simulink model "Modelo_motor_blockset"  (R2023b)
settings: Solver=VariableStepAuto  StartTime=0.0  StopTime=4  RelTol=1e-3
libraries: spsAsynchronousMachineSIUnitsLib x5, simulink x5, spsThreePhaseVIMeasurementLib x5, spsPWMGenerator2LevelLib x4, spsUniversalBridgeLib x4, spsDCVoltageSourceLib x3, spsControlledVoltageSourceLib x1, spsGroundLib x1, spsSVPWMGenerator2LevelLib x1, spsThreePhaseProgrammableVoltageSourceLib x1, sps_lib x1
settings Model: Creator=Jorge  LastModifiedBy=Jorge

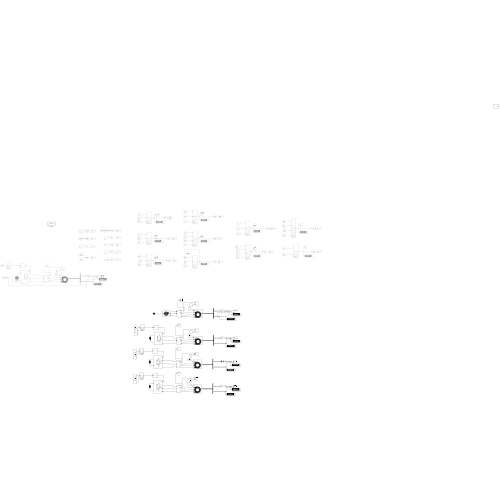
[thumbnail: Simulink's stored preview of the top-level diagram]
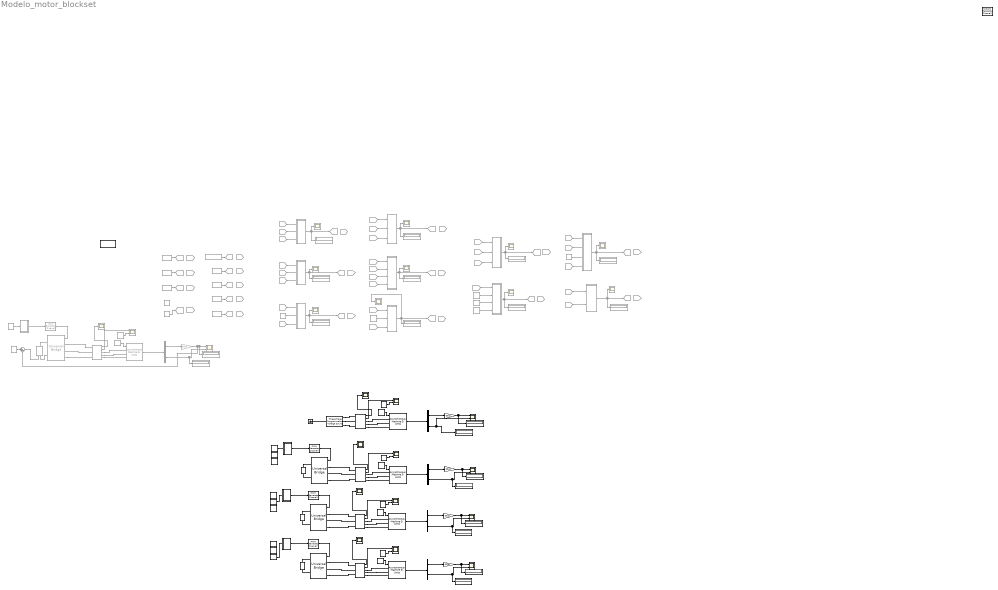
== system Modelo_motor_blockset ==
  120 : Constant  Commented=on  Value=120
  Asynchronous Machine SI Units : spsAsynchronousMachineSIUnitsLib/Asynchronous Machine SI Units  RotorType=Squirrel-cage  PresetModel=No  MechanicalLoad=Torque Tm  ShowDetailedParameters=on  ReferenceFrame=Rotor  Units=SI  MeasurementBus=off  NominalParameters=[950 220 60]  VoltageRatio=1  Stator=[0.2 3/(2*pi*60)]  Rotor=[1.3 2/(2*pi*60)]  Cage1=[0.4155 0.002066]  Cage2=[0.4168 0.0003495]  Lm=28/(2*pi*60)  Mechanical=[0.1 0.0 4]  PolePairs=2  InitialConditions=[1 0 0 0 0 0 120 -120]  SimulateSaturation=off  Saturation=[14.03593122, 27.81365428, 53.79336849, 72.68890987, 97.98006896, 148.6815601, 215.7428561, 302.9841135, 428.7778367 ; 230, 322, 414, 460, 506, 552, 598, 644, 690]  LoadFlowParameters=1492000  TsPowergui=0  TsBlock=-1  IterativeModel=Trapezoidal non iterative  IterativeDiscreteModel=Trapezoidal non iterative  Pmec=866
  Asynchronous Machine SI Units1 : spsAsynchronousMachineSIUnitsLib/Asynchronous Machine SI Units  RotorType=Squirrel-cage  PresetModel=No  MechanicalLoad=Torque Tm  ShowDetailedParameters=on  ReferenceFrame=Rotor  Units=SI  MeasurementBus=off  NominalParameters=[907 220/sqrt(3) 60]  VoltageRatio=1  Stator=[0.2 3/(2*pi*60)]  Rotor=[1.3 2/(2*pi*60)]  Cage1=[0.4155 0.002066]  Cage2=[0.4168 0.0003495]  Lm=28/(2*pi*60)  Mechanical=[0.1 0.0 4]  PolePairs=2  InitialConditions=[1 0 0 0 0 0 -120 120]  SimulateSaturation=off  Saturation=[14.03593122, 27.81365428, 53.79336849, 72.68890987, 97.98006896, 148.6815601, 215.7428561, 302.9841135, 428.7778367 ; 230, 322, 414, 460, 506, 552, 598, 644, 690]  LoadFlowParameters=1492000  TsPowergui=0  TsBlock=-1  IterativeModel=Trapezoidal non iterative  IterativeDiscreteModel=Trapezoidal non iterative  Pmec=866
  Asynchronous Machine SI Units2 : spsAsynchronousMachineSIUnitsLib/Asynchronous Machine SI Units  Commented=on  RotorType=Squirrel-cage  PresetModel=No  MechanicalLoad=Torque Tm  ShowDetailedParameters=on  ReferenceFrame=Rotor  Units=SI  MeasurementBus=off  NominalParameters=[907 220/sqrt(3) 60]  VoltageRatio=1  Stator=[0.2 3/(2*pi*60)]  Rotor=[1.3 2/(2*pi*60)]  Cage1=[0.4155 0.002066]  Cage2=[0.4168 0.0003495]  Lm=28/(2*pi*60)  Mechanical=[0.1 0.0 4]  PolePairs=2  InitialConditions=[1 0 0 0 0 0 -120 120]  SimulateSaturation=off  Saturation=[14.03593122, 27.81365428, 53.79336849, 72.68890987, 97.98006896, 148.6815601, 215.7428561, 302.9841135, 428.7778367 ; 230, 322, 414, 460, 506, 552, 598, 644, 690]  LoadFlowParameters=1492000  TsPowergui=0  TsBlock=-1  IterativeModel=Trapezoidal non iterative  IterativeDiscreteModel=Trapezoidal non iterative  Pmec=866
  Asynchronous Machine SI Units3 : spsAsynchronousMachineSIUnitsLib/Asynchronous Machine SI Units  RotorType=Squirrel-cage  PresetModel=No  MechanicalLoad=Torque Tm  ShowDetailedParameters=on  ReferenceFrame=Rotor  Units=SI  MeasurementBus=off  NominalParameters=[907 220/sqrt(3) 60]  VoltageRatio=1  Stator=[0.2 3/(2*pi*60)]  Rotor=[1.3 2/(2*pi*60)]  Cage1=[0.4155 0.002066]  Cage2=[0.4168 0.0003495]  Lm=28/(2*pi*60)  Mechanical=[0.1 0.0 4]  PolePairs=2  InitialConditions=[1 0 0 0 0 0 -120 120]  SimulateSaturation=off  Saturation=[14.03593122, 27.81365428, 53.79336849, 72.68890987, 97.98006896, 148.6815601, 215.7428561, 302.9841135, 428.7778367 ; 230, 322, 414, 460, 506, 552, 598, 644, 690]  LoadFlowParameters=1492000  TsPowergui=0  TsBlock=-1  IterativeModel=Trapezoidal non iterative  IterativeDiscreteModel=Trapezoidal non iterative  Pmec=866
  Asynchronous Machine SI Units4 : spsAsynchronousMachineSIUnitsLib/Asynchronous Machine SI Units  RotorType=Squirrel-cage  PresetModel=No  MechanicalLoad=Torque Tm  ShowDetailedParameters=on  ReferenceFrame=Rotor  Units=SI  MeasurementBus=off  NominalParameters=[907 220/sqrt(3) 60]  VoltageRatio=1  Stator=[0.2 3/(2*pi*60)]  Rotor=[1.3 2/(2*pi*60)]  Cage1=[0.4155 0.002066]  Cage2=[0.4168 0.0003495]  Lm=28/(2*pi*60)  Mechanical=[0.1 0.0 4]  PolePairs=2  InitialConditions=[1 0 0 0 0 0 -120 120]  SimulateSaturation=off  Saturation=[14.03593122, 27.81365428, 53.79336849, 72.68890987, 97.98006896, 148.6815601, 215.7428561, 302.9841135, 428.7778367 ; 230, 322, 414, 460, 506, 552, 598, 644, 690]  LoadFlowParameters=1492000  TsPowergui=0  TsBlock=-1  IterativeModel=Trapezoidal non iterative  IterativeDiscreteModel=Trapezoidal non iterative  Pmec=866
  Bus Selector{,1,3..4} (4 alike) : BusSelector  OutputSignals=Mechanical.Rotor speed (wm),Mechanical.Electromagnetic torque Te (N*m)
  Bus Selector2 : BusSelector  Commented=on  OutputSignals=Mechanical.Rotor speed (wm),Mechanical.Electromagnetic torque Te (N*m)
  Constant : Constant  Commented=on
  Constant1 : Constant  Commented=on
  Constant{6,10,16,21} (4 alike) : Constant  Value=4.94
  Constant11 : Constant  Commented=on  Value=60
  Constant12 : Constant  Commented=on  Value=4.74
  Constant13 : Constant  Commented=on  Value=1746
  Constant14 : Constant  Value=40
  Constant15 : Constant  Value=20
  Constant17 : Constant  Value=40
  Constant18 : Constant  Value=20
  Constant19 : Constant  Value=60
  Constant2 : Constant  Commented=on  Value=2
  Constant{5,9,20,25} (4 alike) : Constant  Value=4.74
  Constant22 : Constant  Value=40
  Constant23 : Constant  Value=20
  Constant24 : Constant  Value=60
  Constant3 : Constant  Commented=on  Value=0.03
  Constant4 : Constant  Commented=on  Value=60
  Constant7 : Constant  Value=60
  Constant8 : Constant  Commented=on  Value=4.94
  Controlled Voltage Source1 : spsControlledVoltageSourceLib/Controlled Voltage Source  Commented=on  Initialize=on  Source_Type=DC  Amplitude=220  Phase=0  Frequency=0  Measurements=None
  DC Voltage Source : spsDCVoltageSourceLib/DC Voltage Source  Amplitude=220*(sqrt(3)/sqrt(2))*0.945  Measurements=Voltage
  DC Voltage Source1 : spsDCVoltageSourceLib/DC Voltage Source  Amplitude=220*(sqrt(3)/sqrt(2))*0.945  Measurements=Voltage
  DC Voltage Source2 : spsDCVoltageSourceLib/DC Voltage Source  Amplitude=220*(sqrt(3)/sqrt(2))*0.945  Measurements=Voltage
  Display{,1..9,14..15} (12 alike) : Display  Commented=on
  Display{10..13,16..19} (8 alike) : Display
  From{,3,12,34} (4 alike) : From  Commented=on  GotoTag=V1
  From1 : From  Commented=on  GotoTag=R1
  From10 : From  Commented=on  GotoTag=I2
  From11 : From  Commented=on  GotoTag=I1
  From13 : From  Commented=on  GotoTag=R1
  From{2,14,33,37} (4 alike) : From  Commented=on  GotoTag=X1
  From{6,15,25,29} (4 alike) : From  Commented=on  GotoTag=R2
  From16 : From  Commented=on  GotoTag=X2
  From{5,17,21,26,30} (5 alike) : From  Commented=on  GotoTag=S
  From18 : From  Commented=on  GotoTag=f
  From19 : From  Commented=on  GotoTag=p
  From20 : From  Commented=on  GotoTag=Ns
  From22 : From  Commented=on  GotoTag=N
  From23 : From  Commented=on  GotoTag=Ns
  From24 : From  Commented=on  GotoTag=I2
  From27 : From  Commented=on  GotoTag=Pag
  From28 : From  Commented=on  GotoTag=I2
  From31 : From  Commented=on  GotoTag=Pmec
  From32 : From  Commented=on  GotoTag=Xm
  From35 : From  Commented=on  GotoTag=Vth
  From36 : From  Commented=on  GotoTag=Xm
  From38 : From  Commented=on  GotoTag=R1
  From39 : From  Commented=on  GotoTag=Rth
  From4 : From  Commented=on  GotoTag=X2
  From40 : From  Commented=on  GotoTag=Ns
  From41 : From  Commented=on  GotoTag=ws
  From42 : From  Commented=on  GotoTag=Pag
  From43 : From  Commented=on  GotoTag=ws
  From44 : From  Commented=on  GotoTag=T
  From7 : From  Commented=on  GotoTag=f
  From8 : From  Commented=on  GotoTag=p
  From9 : From  Commented=on  GotoTag=Xm
  Gain{,2..4} (4 alike) : Gain  Gain=60/pi
  Gain1 : Gain  Commented=on  Gain=60/pi
  Goto : Goto  Commented=on  GotoTag=V1
  Goto1 : Goto  Commented=on  GotoTag=f
  Goto10 : Goto  Commented=on  GotoTag=I1
  Goto11 : Goto  Commented=on  GotoTag=Ns
  Goto12 : Goto  Commented=on  GotoTag=N
  Goto13 : Goto  Commented=on  GotoTag=Pag
  Goto14 : Goto  Commented=on  GotoTag=Pmec
  Goto15 : Goto  Commented=on  GotoTag=Vth
  Goto16 : Goto  Commented=on  GotoTag=Rth
  Goto17 : Goto  Commented=on  GotoTag=ws
  Goto18 : Goto  Commented=on  GotoTag=T
  Goto2 : Goto  Commented=on  GotoTag=p
  Goto3 : Goto  Commented=on  GotoTag=R1
  Goto4 : Goto  Commented=on  GotoTag=X1
  Goto5 : Goto  Commented=on  GotoTag=R2
  Goto6 : Goto  Commented=on  GotoTag=X2
  Goto7 : Goto  Commented=on  GotoTag=Xm
  Goto8 : Goto  Commented=on  GotoTag=S
  Goto9 : Goto  Commented=on  GotoTag=I2
  Ground : spsGroundLib/Ground  LConnTagsString=a
  PWM Generator (2-Level) : spsPWMGenerator2LevelLib/PWM Generator (2-Level)  ModulatorType=Three-phase bridge (6 pulses)  ModulatorMode=Unsynchronized  Fc=60*39  Pc=0  nF=27  MinMax="[ -1  1 ]"  SamplingTechnique=Natural  ModulatingSignals=off  m=0.8  Freq=60  Phase=0  Ts=0  ShowCarrierOutport=off
  PWM Generator (2-Level)1 : spsPWMGenerator2LevelLib/PWM Generator (2-Level)  Commented=on  ModulatorType=Three-phase bridge (6 pulses)  ModulatorMode=Unsynchronized  Fc=60*39  Pc=0  nF=27  MinMax="[ -1  1 ]"  SamplingTechnique=Natural  ModulatingSignals=off  m=0.8  Freq=60  Phase=0  Ts=0  ShowCarrierOutport=off
  PWM Generator (2-Level)2 : spsPWMGenerator2LevelLib/PWM Generator (2-Level)  ModulatorType=Three-phase bridge (6 pulses)  ModulatorMode=Unsynchronized  Fc=60*39  Pc=0  nF=27  MinMax="[ -1  1 ]"  SamplingTechnique=Natural  ModulatingSignals=off  m=0.8  Freq=60  Phase=0  Ts=0  ShowCarrierOutport=off
  PWM Generator (2-Level)3 : spsPWMGenerator2LevelLib/PWM Generator (2-Level)  ModulatorType=Three-phase bridge (6 pulses)  ModulatorMode=Unsynchronized  Fc=60*39  Pc=0  nF=27  MinMax="[ -1  1 ]"  SamplingTechnique=Natural  ModulatingSignals=off  m=0.8  Freq=60  Phase=0  Ts=0  ShowCarrierOutport=off
  Pi : Constant  Commented=on  Value=pi  OutDataTypeStr=Inherit: Inherit via back propagation
  R1 : Constant  Commented=on  Value=0.2
  R2 : Constant  Commented=on  Value=1.3
  SVPWM Generator (2-Level) : spsSVPWMGenerator2LevelLib/SVPWM Generator (2-Level)  InputType=Internally generated  SwitchingPattern=Pattern #1  Fc=2000  ParUref=[1 0 60]  Ts=0
  Scope{,1..9,17} (11 alike) : Scope  Commented=on
  Scope{10..11,13,15,19,21..22,24} (8 alike) : Scope  NumInputPorts=2
  Scope{12,14,20,23} (4 alike) : Scope
  Scope16 : Scope  Commented=on  NumInputPorts=2
  Scope18 : Scope  Commented=on  NumInputPorts=2
  Sinal : Subsystem
  Sinal1 : Subsystem  Commented=on
  Sinal2 : Subsystem
  Sinal3 : Subsystem
  Subsystem : Subsystem  Commented=on
  Subsystem1 : Subsystem  Commented=on
  Subsystem2 : Subsystem  Commented=on
  Subsystem3 : Subsystem  Commented=on
  Subsystem4 : Subsystem  Commented=on
  Subsystem5 : Subsystem  Commented=on
  Subsystem6 : Subsystem  Commented=on
  Subsystem7 : Subsystem  Commented=on
  Subsystem8 : Subsystem  Commented=on
  Subsystem9 : Subsystem  Commented=on
  Sum : Sum  Commented=on  Inputs=|+-
  Three-Phase Programmable Voltage Source : spsThreePhaseProgrammableVoltageSourceLib/Three-Phase Programmable Voltage Source  PositiveSequence=[220/sqrt(2) 0 60]  VariationEntity=None  VariationType=Table of time-amplitude pairs  VariationTypeAlt=Step  VariationStep=0.5  VariationRate=10  VariationMagnitude=0.3  VariationFrequency=2  VariationTiming=[1 2]  VariationPhaseA=off  Amplitudes=[1 0.8 1.2 1.0]  TimeValues=[0 0.1 0.15 0.2]  HarmonicGeneration=off  HarmonicA=[3 0.2 -25 0]  HarmonicB=[2 0.15 35 2]  Timing="[0.05  3]"  BusType=swing  Pref=0  Qref=0  Qmin=-inf  Qmax=inf
  Three-Phase V-I Measurement{,1,3..4} (4 alike) : spsThreePhaseVIMeasurementLib/Three-Phase V-I Measurement  VoltageMeasurement=phase-to-phase  SetLabelV=off  LabelV=Vabc  Vpu=off  VpuLL=off  CurrentMeasurement=yes  SetLabelI=off  LabelI=Iabc  Ipu=off  Pbase=100e6  Vbase=500e3  OutputType=Complex  PhasorSimulation=off  PSBequivalent=0
  Three-Phase V-I Measurement2 : spsThreePhaseVIMeasurementLib/Three-Phase V-I Measurement  Commented=on  VoltageMeasurement=phase-to-phase  SetLabelV=off  LabelV=Vabc  Vpu=off  VpuLL=off  CurrentMeasurement=yes  SetLabelI=off  LabelI=Iabc  Ipu=off  Pbase=100e6  Vbase=500e3  OutputType=Complex  PhasorSimulation=off  PSBequivalent=0
  Universal Bridge : spsUniversalBridgeLib/Universal Bridge  Arms=3  SnubberResistance=1e5  SnubberCapacitance=inf  Device=IGBT / Diodes  Ron=1e-3  Lon=0  ForwardVoltages="[  0  0  ]"  ForwardVoltage=0  GTOparameters=[ 10e-6 , 20e-6 ]  IGBTparameters=[ 1e-6 , 2e-6 ]  Measurements=None  Measurements_2=None  converterType=Rectifier
  Universal Bridge1 : spsUniversalBridgeLib/Universal Bridge  Commented=on  Arms=3  SnubberResistance=1e5  SnubberCapacitance=inf  Device=IGBT / Diodes  Ron=1e-3  Lon=0  ForwardVoltages="[  0  0  ]"  ForwardVoltage=0  GTOparameters=[ 10e-6 , 20e-6 ]  IGBTparameters=[ 1e-6 , 2e-6 ]  Measurements=None  Measurements_2=None  converterType=Rectifier
  Universal Bridge2 : spsUniversalBridgeLib/Universal Bridge  Arms=3  SnubberResistance=1e5  SnubberCapacitance=inf  Device=IGBT / Diodes  Ron=1e-3  Lon=0  ForwardVoltages="[  0  0  ]"  ForwardVoltage=0  GTOparameters=[ 10e-6 , 20e-6 ]  IGBTparameters=[ 1e-6 , 2e-6 ]  Measurements=None  Measurements_2=None  converterType=Rectifier
  Universal Bridge3 : spsUniversalBridgeLib/Universal Bridge  Arms=3  SnubberResistance=1e5  SnubberCapacitance=inf  Device=IGBT / Diodes  Ron=1e-3  Lon=0  ForwardVoltages="[  0  0  ]"  ForwardVoltage=0  GTOparameters=[ 10e-6 , 20e-6 ]  IGBTparameters=[ 1e-6 , 2e-6 ]  Measurements=None  Measurements_2=None  converterType=Rectifier
  V1 : Constant  Commented=on  Value=220*sqrt(2)/sqrt(3)
  X1 : Constant  Commented=on  Value=0.0079
  X2 : Constant  Commented=on  Value=0.0053
  Xm : Constant  Commented=on  Value=28
  escorregamento : simulink/Sources/Ramp  Commented=on  slope=-0.01  start=0  InitialOutput=1
  f : Constant  Commented=on  Value=60
  p : Constant  Commented=on  Value=4
  powergui : sps_lib/powergui  Priority=1  SimulationMode=Continuous  SampleTime=50e-6  frequency=60  Iterations=50  frequencyindice=60  Pbase=100e6  ErrMax=1e-4  UnitsV=kV  UnitsW=MW  buscounter=0  FunctionMessages=off  echomessages=off  EnableUseOfTLC=off  CurrentSourceSwitches=off  DisableSnubberDevices=off  DisableRonSwitches=off  DisableVfSwitches=off  DisplayEquations=off  AutomaticDiscreteSolvers=off  SolverType=Tustin/Backward Euler (TBE)  Interpol=off  ExternalGateDelay=off  methode=off  Ts=100  x0status=blocks  SPID=on  SwTol=0  HookPort=off  NonlinearTolerance=1e-4  nMaxIteration=100  ContinueOnMaxIteration=off  RestoreLinks=warning  ResistiveCurrentMeasurement=off  Frange=[0:2:500]  Ylog=off  Xlog=on  ShowGrid=off  save=off  variable=ZData  structure=0  ZoomFFT=off  StartTime=0.0  cycles=1  DisplayStyle=1  fundamental=60  FreqAxis=off  MaxFrequency=1000  frequencyindicesteady=1  RmsSteady=1  display=off
  wires:
  V1/1 -> Goto/1
  f/1 -> Goto1/1
  p/1 -> Goto2/1
  R1/1 -> Goto3/1
  X1/1 -> Goto4/1
  R2/1 -> Goto5/1
  X2/1 -> Goto6/1
  Xm/1 -> Goto7/1
  From/1 -> Subsystem/1(In1)
  From1/1 -> Subsystem/2(In2)
  From2/1 -> Subsystem/3(In3)
  Subsystem/1(I1) -> Goto10/1, Scope/1, Display/1
  Subsystem1/1(I2) -> Goto9/1, Display1/1, Scope1/1
  From6/1 -> Subsystem1/2(In2)
  From4/1 -> Subsystem1/4(In4)
  From20/1 -> Subsystem2/1(In1)
  Constant/1 -> Subsystem2/2(In2)
  From21/1 -> Subsystem2/3(In3)
  Subsystem2/1(Out1) -> Scope3/1, Display3/1, Goto12/1  "N"
  From24/1 -> Subsystem3/1(In1)
  From25/1 -> Subsystem3/2(In2)
  Subsystem3/1(Pag) -> Scope4/1, Display4/1, Goto13/1
  From28/1 -> Subsystem4/1(In1)
  From29/1 -> Subsystem4/2(In2)
  Constant1/1 -> Subsystem4/3(In3)
  From30/1 -> Subsystem4/4(In4)
  Subsystem4/1(Pmec) -> Display5/1, Goto14/1, Scope5/1
  Subsystem5/1(Ns) -> Display2/1, Scope2/1, Goto11/1
  From18/1 -> Subsystem5/1(In1)
  120/1 -> Subsystem5/2(In2)
  From19/1 -> Subsystem5/3(In3)
  Subsystem6/1(Out1) -> Scope6/1, Goto15/1, Display6/1  "Vth"
  From34/1 -> Subsystem6/1(In1)
  From33/1 -> Subsystem6/2(In2)
  From32/1 -> Subsystem6/3(In3)
  From38/1 -> Subsystem7/1(In1)
  From37/1 -> Subsystem7/2(In2)
  From36/1 -> Subsystem7/3(In3)
  Subsystem7/1(Rth) -> Display7/1, Scope7/1, Goto16/1
  From40/1 -> Subsystem8/1(In1)
  Constant2/1 -> Subsystem8/2(In2)
  Pi/1 -> Subsystem8/3(In3)
  Constant4/1 -> Subsystem8/4(In4)
  Subsystem8/1(Out1) -> Scope8/1, Display8/1, Goto17/1
  Subsystem9/1(Out1) -> Scope9/1, Display9/1, Goto18/1  "T"
  From42/1 -> Subsystem9/1(In1)
  From43/1 -> Subsystem9/2(In2)
  From26/1 -> Subsystem3/3(In3)
  From5/1 -> Subsystem1/3(In3)
  From3/1 -> Subsystem1/1(In1)
  Three-Phase V-I Measurement/1 -> Scope12/1
  Three-Phase V-I Measurement/2 -> Scope11/1
  Asynchronous Machine SI Units/1 -> Bus Selector/1
  Constant3/1 -> Goto8/1
  Bus Selector/1 -> Gain/1  "<Rotor speed (wm)>"
  Bus Selector/2 -> Display10/1, Scope13/2  "<Electromagnetic torque Te (N*m)>"
  Gain/1 -> Display12/1, Scope13/1  "Velocidade (RPM)"
  Constant5/1 -> Asynchronous Machine SI Units/1
  Constant6/1 -> Scope11/2
  Constant10/1 -> Scope10/2
  Asynchronous Machine SI Units1/1 -> Bus Selector1/1
  Gain3/1 -> Display13/1, Scope15/1  "Velocidade (RPM)"
  Three-Phase V-I Measurement1/1 -> Scope14/1
  Bus Selector1/2 -> Display11/1, Scope15/2  "<Electromagnetic torque Te (N*m)>"
  Constant9/1 -> Asynchronous Machine SI Units1/1
  Bus Selector1/1 -> Gain3/1  "<Rotor speed (wm)>"
  Three-Phase V-I Measurement1/2 -> Scope10/1
  PWM Generator (2-Level)/1 -> Universal Bridge/1
  Sinal/1(Out1) -> PWM Generator (2-Level)/1
  Sinal1/1(Out1) -> PWM Generator (2-Level)1/1
  Sum/1 -> Controlled Voltage Source1/1
  Three-Phase V-I Measurement2/1 -> Scope17/1
  PWM Generator (2-Level)1/1 -> Universal Bridge1/1
  Constant11/1 -> Sinal1/1(In1)
  Constant12/1 -> Asynchronous Machine SI Units2/1
  Bus Selector2/2 -> Display14/1, Scope18/2  "<Electromagnetic torque Te (N*m)>"
  Three-Phase V-I Measurement2/2 -> Scope16/1
  Asynchronous Machine SI Units2/1 -> Bus Selector2/1
  Constant8/1 -> Scope16/2
  Bus Selector2/1 -> Gain1/1  "<Rotor speed (wm)>"
  Gain1/1 -> Sum/2, Display15/1, Scope18/1  "Velocidade (RPM)"
  Constant13/1 -> Sum/1
  Sinal2/1(Out1) -> PWM Generator (2-Level)2/1
  PWM Generator (2-Level)2/1 -> Universal Bridge2/1
  Three-Phase V-I Measurement3/2 -> Scope19/1
  Bus Selector3/1 -> Gain2/1  "<Rotor speed (wm)>"
  Constant20/1 -> Asynchronous Machine SI Units3/1
  Bus Selector3/2 -> Scope21/2, Display16/1  "<Electromagnetic torque Te (N*m)>"
  Three-Phase V-I Measurement3/1 -> Scope20/1
  Gain2/1 -> Scope21/1, Display17/1  "Velocidade (RPM)"
  Asynchronous Machine SI Units3/1 -> Bus Selector3/1
  Constant16/1 -> Scope19/2
  Constant21/1 -> Scope22/2
  Asynchronous Machine SI Units4/1 -> Bus Selector4/1
  Gain4/1 -> Display19/1, Scope24/1  "Velocidade (RPM)"
  Three-Phase V-I Measurement4/1 -> Scope23/1
  Bus Selector4/2 -> Display18/1, Scope24/2  "<Electromagnetic torque Te (N*m)>"
  Constant25/1 -> Asynchronous Machine SI Units4/1
  Bus Selector4/1 -> Gain4/1  "<Rotor speed (wm)>"
  Three-Phase V-I Measurement4/2 -> Scope22/1
  PWM Generator (2-Level)3/1 -> Universal Bridge3/1
  Sinal3/1(Out1) -> PWM Generator (2-Level)3/1
  Constant17/1 -> Sinal2/1(In1)
  Constant7/1 -> Sinal/1(In1)
  Constant23/1 -> Sinal3/1(In1)
  connections:
  Three-Phase Programmable Voltage Source/LConn1 -- Ground/LConn1
  Three-Phase V-I Measurement/RConn1 -- Asynchronous Machine SI Units/LConn1
  Three-Phase V-I Measurement/RConn2 -- Asynchronous Machine SI Units/LConn2
  Three-Phase V-I Measurement/RConn3 -- Asynchronous Machine SI Units/LConn3
  Three-Phase Programmable Voltage Source/RConn1 -- Three-Phase V-I Measurement/LConn1
  Three-Phase Programmable Voltage Source/RConn2 -- Three-Phase V-I Measurement/LConn2
  Three-Phase Programmable Voltage Source/RConn3 -- Three-Phase V-I Measurement/LConn3
  DC Voltage Source/RConn1 -- Universal Bridge/RConn1
  Universal Bridge/RConn2 -- DC Voltage Source/LConn1
  Universal Bridge/LConn3 -- Three-Phase V-I Measurement1/LConn3
  Three-Phase V-I Measurement1/LConn2 -- Universal Bridge/LConn2
  Three-Phase V-I Measurement1/RConn3 -- Asynchronous Machine SI Units1/LConn3
  Universal Bridge/LConn1 -- Three-Phase V-I Measurement1/LConn1
  Three-Phase V-I Measurement1/RConn2 -- Asynchronous Machine SI Units1/LConn2
  Three-Phase V-I Measurement1/RConn1 -- Asynchronous Machine SI Units1/LConn1
  Universal Bridge1/LConn1 -- Three-Phase V-I Measurement2/LConn1
  Universal Bridge1/RConn2 -- Controlled Voltage Source1/LConn1
  Three-Phase V-I Measurement2/LConn2 -- Universal Bridge1/LConn2
  Controlled Voltage Source1/RConn1 -- Universal Bridge1/RConn1
  Three-Phase V-I Measurement2/RConn1 -- Asynchronous Machine SI Units2/LConn1
  Universal Bridge1/LConn3 -- Three-Phase V-I Measurement2/LConn3
  Three-Phase V-I Measurement2/RConn3 -- Asynchronous Machine SI Units2/LConn3
  Three-Phase V-I Measurement2/RConn2 -- Asynchronous Machine SI Units2/LConn2
  Three-Phase V-I Measurement3/RConn1 -- Asynchronous Machine SI Units3/LConn1
  Three-Phase V-I Measurement3/RConn2 -- Asynchronous Machine SI Units3/LConn2
  Universal Bridge2/LConn1 -- Three-Phase V-I Measurement3/LConn1
  Universal Bridge2/LConn3 -- Three-Phase V-I Measurement3/LConn3
  Universal Bridge2/RConn2 -- DC Voltage Source1/LConn1
  DC Voltage Source1/RConn1 -- Universal Bridge2/RConn1
  Three-Phase V-I Measurement3/LConn2 -- Universal Bridge2/LConn2
  Three-Phase V-I Measurement3/RConn3 -- Asynchronous Machine SI Units3/LConn3
  Three-Phase V-I Measurement4/LConn2 -- Universal Bridge3/LConn2
  Universal Bridge3/LConn3 -- Three-Phase V-I Measurement4/LConn3
  Universal Bridge3/RConn2 -- DC Voltage Source2/LConn1
  Universal Bridge3/LConn1 -- Three-Phase V-I Measurement4/LConn1
  DC Voltage Source2/RConn1 -- Universal Bridge3/RConn1
  Three-Phase V-I Measurement4/RConn2 -- Asynchronous Machine SI Units4/LConn2
  Three-Phase V-I Measurement4/RConn1 -- Asynchronous Machine SI Units4/LConn1
  Three-Phase V-I Measurement4/RConn3 -- Asynchronous Machine SI Units4/LConn3

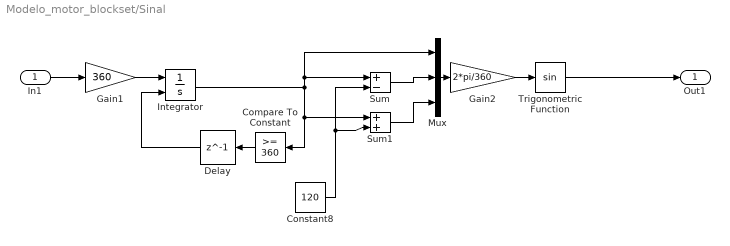
== system Modelo_motor_blockset/Sinal ==
  In1 : Inport
  Compare To Constant : simulink/Logic and Bit Operations/Compare To Constant  relop=>=  const=360  OutDataTypeStr=boolean
  Constant8 : Constant  Value=120
  Delay : Delay  DelayLength=1
  Gain1 : Gain  Gain=360
  Gain2 : Gain  Gain=2*pi/360
  Integrator : Integrator  ExternalReset=rising
  Mux : Mux  Inputs=3
  Sum : Sum  Inputs=+-
  Sum1 : Sum
  Trigonometric Function : Trigonometry
  Out1 : Outport
  wires:
  Sum/1 -> Mux/2
  Constant8/1 -> Sum1/2, Sum/2
  Gain1/1 -> Integrator/1
  Integrator/1 -> Sum1/1, Compare To Constant/1, Mux/1, Sum/1
  In1/1 -> Gain1/1
  Gain2/1 -> Trigonometric Function/1
  Trigonometric Function/1 -> Out1/1
  Mux/1 -> Gain2/1
  Delay/1 -> Integrator/2
  Compare To Constant/1 -> Delay/1
  Sum1/1 -> Mux/3

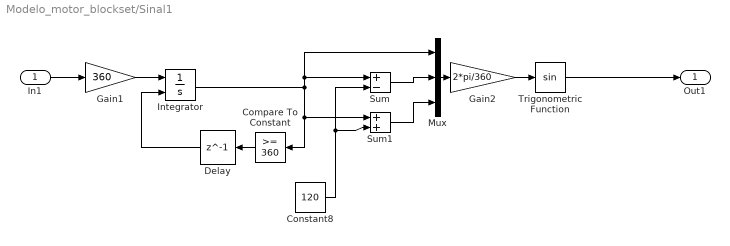
== system Modelo_motor_blockset/Sinal1 ==
  In1 : Inport
  Compare To Constant : simulink/Logic and Bit Operations/Compare To Constant  relop=>=  const=360  OutDataTypeStr=boolean
  Constant8 : Constant  Value=120
  Delay : Delay  DelayLength=1
  Gain1 : Gain  Gain=360
  Gain2 : Gain  Gain=2*pi/360
  Integrator : Integrator  ExternalReset=rising
  Mux : Mux  Inputs=3
  Sum : Sum  Inputs=+-
  Sum1 : Sum
  Trigonometric Function : Trigonometry
  Out1 : Outport
  wires:
  Sum/1 -> Mux/2
  Constant8/1 -> Sum1/2, Sum/2
  Gain1/1 -> Integrator/1
  Integrator/1 -> Sum1/1, Compare To Constant/1, Mux/1, Sum/1
  In1/1 -> Gain1/1
  Gain2/1 -> Trigonometric Function/1
  Trigonometric Function/1 -> Out1/1
  Mux/1 -> Gain2/1
  Delay/1 -> Integrator/2
  Compare To Constant/1 -> Delay/1
  Sum1/1 -> Mux/3

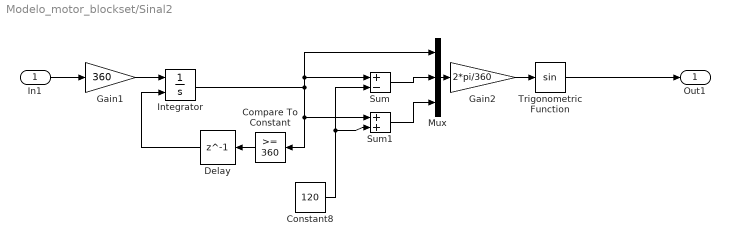
== system Modelo_motor_blockset/Sinal2 ==
  In1 : Inport
  Compare To Constant : simulink/Logic and Bit Operations/Compare To Constant  relop=>=  const=360  OutDataTypeStr=boolean
  Constant8 : Constant  Value=120
  Delay : Delay  DelayLength=1
  Gain1 : Gain  Gain=360
  Gain2 : Gain  Gain=2*pi/360
  Integrator : Integrator  ExternalReset=rising
  Mux : Mux  Inputs=3
  Sum : Sum  Inputs=+-
  Sum1 : Sum
  Trigonometric Function : Trigonometry
  Out1 : Outport
  wires:
  Sum1/1 -> Mux/3
  Compare To Constant/1 -> Delay/1
  Delay/1 -> Integrator/2
  Mux/1 -> Gain2/1
  Trigonometric Function/1 -> Out1/1
  Gain2/1 -> Trigonometric Function/1
  In1/1 -> Gain1/1
  Integrator/1 -> Sum/1, Mux/1, Compare To Constant/1, Sum1/1
  Gain1/1 -> Integrator/1
  Constant8/1 -> Sum/2, Sum1/2
  Sum/1 -> Mux/2

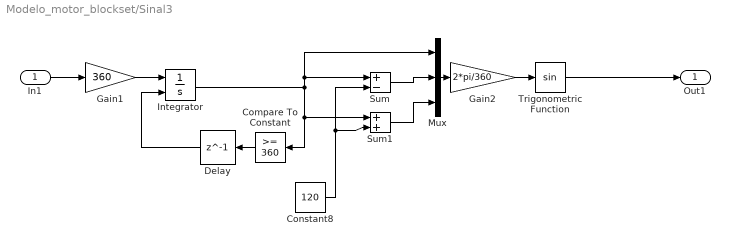
== system Modelo_motor_blockset/Sinal3 ==
  In1 : Inport
  Compare To Constant : simulink/Logic and Bit Operations/Compare To Constant  relop=>=  const=360  OutDataTypeStr=boolean
  Constant8 : Constant  Value=120
  Delay : Delay  DelayLength=1
  Gain1 : Gain  Gain=360
  Gain2 : Gain  Gain=2*pi/360
  Integrator : Integrator  ExternalReset=rising
  Mux : Mux  Inputs=3
  Sum : Sum  Inputs=+-
  Sum1 : Sum
  Trigonometric Function : Trigonometry
  Out1 : Outport
  wires:
  Sum/1 -> Mux/2
  Constant8/1 -> Sum1/2, Sum/2
  Gain1/1 -> Integrator/1
  Integrator/1 -> Sum1/1, Compare To Constant/1, Mux/1, Sum/1
  In1/1 -> Gain1/1
  Gain2/1 -> Trigonometric Function/1
  Trigonometric Function/1 -> Out1/1
  Mux/1 -> Gain2/1
  Delay/1 -> Integrator/2
  Compare To Constant/1 -> Delay/1
  Sum1/1 -> Mux/3

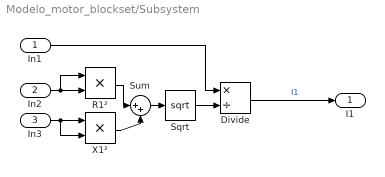
== system Modelo_motor_blockset/Subsystem ==
  In1 : Inport
  In2 : Inport  Port=2
  In3 : Inport  Port=3
  Divide : Product  Inputs=*/
  R1² : Product
  Sqrt : Sqrt
  Sum : Sum  Inputs=|++
  X1² : Product
  I1 : Outport
  wires:
  In3/1 -> X1²/2, X1²/1
  Divide/1 -> I1/1  "I1"
  In2/1 -> R1²/1, R1²/2
  Sqrt/1 -> Divide/2
  R1²/1 -> Sum/1
  Sum/1 -> Sqrt/1
  X1²/1 -> Sum/2
  In1/1 -> Divide/1

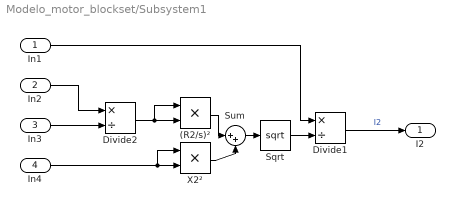
== system Modelo_motor_blockset/Subsystem1 ==
  In1 : Inport
  In2 : Inport  Port=2
  In3 : Inport  Port=3
  In4 : Inport  Port=4
  (R2/s)² : Product
  Divide1 : Product  Inputs=*/
  Divide2 : Product  Inputs=*/
  Sqrt : Sqrt
  Sum : Sum  Inputs=|++
  X2² : Product
  I2 : Outport
  wires:
  Sqrt/1 -> Divide1/2
  X2²/1 -> Sum/2
  Divide2/1 -> (R2/s)²/1, (R2/s)²/2
  Sum/1 -> Sqrt/1
  In2/1 -> Divide2/1
  (R2/s)²/1 -> Sum/1
  In4/1 -> X2²/1, X2²/2
  In1/1 -> Divide1/1
  In3/1 -> Divide2/2
  Divide1/1 -> I2/1  "I2"

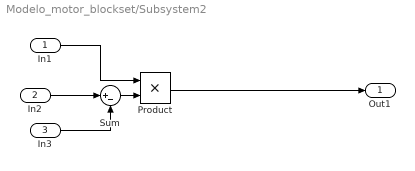
== system Modelo_motor_blockset/Subsystem2 ==
  In1 : Inport
  In2 : Inport  Port=2
  In3 : Inport  Port=3
  Product : Product
  Sum : Sum  Inputs=|+-
  Out1 : Outport
  wires:
  In1/1 -> Product/1
  Sum/1 -> Product/2
  In3/1 -> Sum/2
  Product/1 -> Out1/1
  In2/1 -> Sum/1

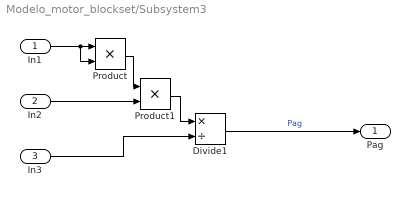
== system Modelo_motor_blockset/Subsystem3 ==
  In1 : Inport
  In2 : Inport  Port=2
  In3 : Inport  Port=3
  Divide1 : Product  Inputs=*/
  Product : Product
  Product1 : Product
  Pag : Outport
  wires:
  Product1/1 -> Divide1/1
  Product/1 -> Product1/1
  In2/1 -> Product1/2
  Divide1/1 -> Pag/1  "Pag"
  In1/1 -> Product/2, Product/1
  In3/1 -> Divide1/2

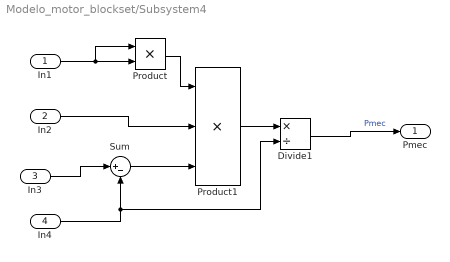
== system Modelo_motor_blockset/Subsystem4 ==
  In1 : Inport
  In2 : Inport  Port=2
  In3 : Inport  Port=3
  In4 : Inport  Port=4
  Divide1 : Product  Inputs=*/
  Product : Product
  Product1 : Product  Inputs=3
  Sum : Sum  Inputs=|+-
  Pmec : Outport
  wires:
  In3/1 -> Sum/1
  Product/1 -> Product1/1
  Sum/1 -> Product1/3
  In1/1 -> Product/2, Product/1
  Divide1/1 -> Pmec/1  "Pmec"
  In4/1 -> Divide1/2, Sum/2
  Product1/1 -> Divide1/1
  In2/1 -> Product1/2

== system Modelo_motor_blockset/Subsystem5 ==
  In1 : Inport
  In2 : Inport  Port=2
  In3 : Inport  Port=3
  Divide : Product  Inputs=**/
  Ns : Outport
  wires:
  In1/1 -> Divide/1
  In2/1 -> Divide/2
  In3/1 -> Divide/3
  Divide/1 -> Ns/1  "Ns"

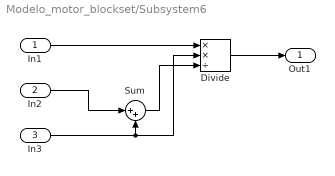
== system Modelo_motor_blockset/Subsystem6 ==
  In1 : Inport
  In2 : Inport  Port=2
  In3 : Inport  Port=3
  Divide : Product  Inputs=**/
  Sum : Sum  Inputs=|++
  Out1 : Outport
  wires:
  In3/1 -> Divide/2, Sum/2
  Sum/1 -> Divide/3
  In2/1 -> Sum/1
  Divide/1 -> Out1/1
  In1/1 -> Divide/1

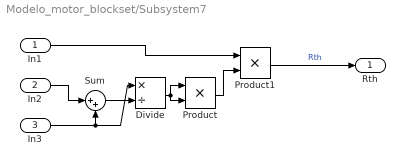
== system Modelo_motor_blockset/Subsystem7 ==
  In1 : Inport
  In2 : Inport  Port=2
  In3 : Inport  Port=3
  Divide : Product  Inputs=*/
  Product : Product
  Product1 : Product
  Sum : Sum  Inputs=|++
  Rth : Outport
  wires:
  Product/1 -> Product1/2
  In1/1 -> Product1/1
  Divide/1 -> Product/1, Product/2
  In3/1 -> Divide/1, Sum/2
  Sum/1 -> Divide/2
  In2/1 -> Sum/1
  Product1/1 -> Rth/1  "Rth"

== system Modelo_motor_blockset/Subsystem8 ==
  In1 : Inport
  In2 : Inport  Port=2
  In3 : Inport  Port=3
  In4 : Inport  Port=4
  Divide : Product  Inputs=***/
  Out1 : Outport
  wires:
  In3/1 -> Divide/3
  In2/1 -> Divide/2
  In4/1 -> Divide/4
  Divide/1 -> Out1/1
  In1/1 -> Divide/1

== system Modelo_motor_blockset/Subsystem9 ==
  In1 : Inport
  In2 : Inport  Port=2
  Divide : Product  Inputs=*/
  Out1 : Outport
  wires:
  Divide/1 -> Out1/1
  In1/1 -> Divide/1
  In2/1 -> Divide/2
